simulink library "csc_snp_sensor_prep_lib"  (R2015b)
settings: Solver=ode45  SolverMode=SingleTasking  StartTime=0.0  StopTime=10.0  RelTol=1e-3
values from neighbouring files (symbols this model uses):
  snp_dtheta_filter_coeffs = fir1(snp_dtheta_filter_order,snp_dtheta_filter_freq)    [csc_snp_sensor_prep_init.m]
  snp_dtheta_filter_order = 1    [csc_snp_sensor_prep_init.m]
  snp_meas_noise_alt = [0.2 1000 1000]    [csc_snp_sensor_prep_init.m]
  snp_meas_noise_angle = 90.0    (= 90)    [csc_snp_sensor_prep_init.m]
  snp_meas_noise_angle_exp = 10    [csc_snp_sensor_prep_init.m]
  snp_meas_noise_angle_gain = 0.0    (= 0)    [csc_snp_sensor_prep_init.m]
  snp_meas_noise_dtheta = 4.0    (= 4)    [csc_snp_sensor_prep_init.m]
  snp_meas_noise_dtheta_exp = 11    [csc_snp_sensor_prep_init.m]
  snp_meas_noise_dtheta_gain = 0.0    (= 0)    [csc_snp_sensor_prep_init.m]
  snp_meas_noise_indep = [ 9e-4 9e-4 9e-4]    [csc_snp_sensor_prep_init.m]
  snp_R_lower_limit_alt = [0.001 10 10 ]    [csc_snp_sensor_prep_init.m]
  snp_R_lower_limit_angle = 0.0001    [csc_snp_sensor_prep_init.m]
  snp_R_lower_limit_dtheta = 0.0001    [csc_snp_sensor_prep_init.m]
  snp_zero_index = zeros(1,kfl_n_meas)    [csc_snp_sensor_prep_init.m]
  snp_zero_meas = zeros(kfl_n_meas,1)    [csc_snp_sensor_prep_init.m]
undefined symbols (not defined in the file or in its folder): kfl_topo_z_to_alt
libraries: simulink x4, util_info_lib x3, csc_hmg_homoraphy_meas_lib x3, csc_imu_sensor_prep_lib x3, csc_rsp_radar_sensor_prep_lib x3, csc_stg_tracker_sensor_prep_lib x3, csu_egm_estimated_gravity_model_lib x3
settings Model: ExtModeAutoUpdateStatusClock=off  Creator=Administrator  LastModifiedBy=Mark Agbayani
settings DataIOCC: SaveFormat=Array  SignalLoggingSaveFormat=ModelDataLogs
settings OptimizationCC: BlockReduction=off  BooleanDataType=off  ExpressionDepthLimit=2147483647
settings DebuggingCC: SaveWithParameterizedLinksMsg=none  UnderspecifiedInitializationDetection=Classic  MergeDetectMultiDrivingBlocksExec=none  SignalResolutionControl=TryResolveAllWithWarning  FcnCallInpInsideContextMsg=EnableAllAsWarning  StateNameClashWarn=warning  StrictBusMsg=Warning
settings HardwareCC: ProdBitPerPointer=32  ProdLargestAtomicFloat=None  ProdIntDivRoundTo=Undefined  ProdEndianess=Unspecified  ProdWordSize=32  ProdHWDeviceType=32-bit Generic  TargetUnknown=on
settings GRTTargetCC: GeneratePreprocessorConditionals=Disable all  CombineOutputUpdateFcns=off  GRTInterface=on
settings ConfigComp: CovModelRefEnable=Off  CovSFcnEnable=off

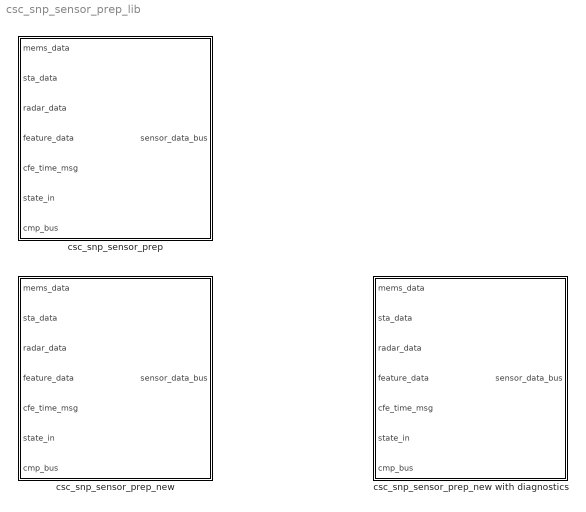
== system csc_snp_sensor_prep_lib ==
  csc_snp_sensor_prep : Subsystem
  csc_snp_sensor_prep_new : Subsystem
  csc_snp_sensor_prep_new with diagnostics : Subsystem  AncestorBlock=csc_snp_sensor_prep_lib/csc_snp_sensor_prep_new

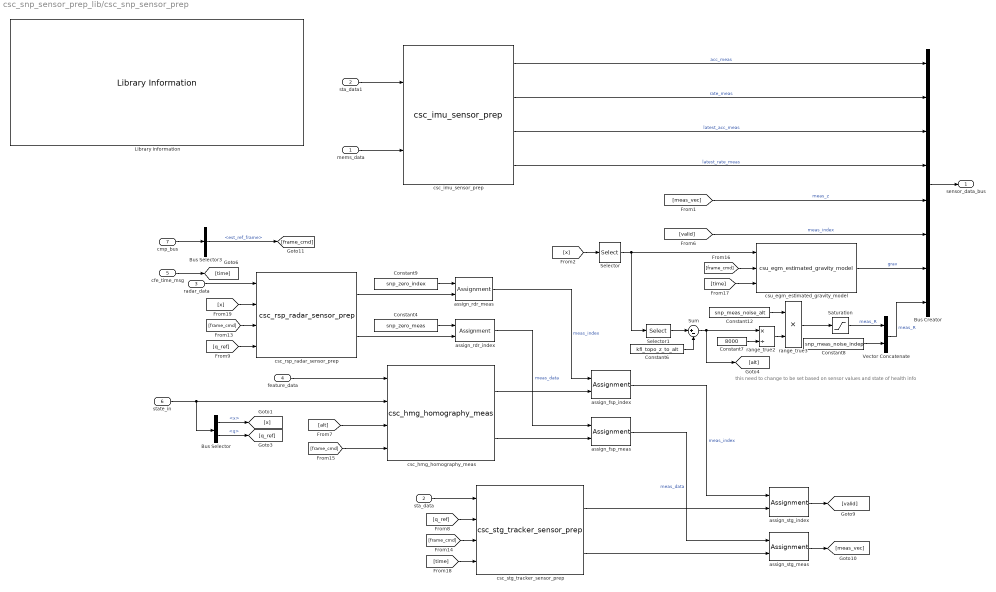
== system csc_snp_sensor_prep_lib/csc_snp_sensor_prep ==
  note: this need to change to be set based on sensor values and state of health info
  mems_data : Inport
  sta_data : Inport  Port=2
  radar_data : Inport  Port=3
  feature_data : Inport  Port=4
  cfe_time_msg : Inport  Port=5
  state_in : Inport  Port=6
  cmp_bus : Inport  Port=7
  Bus Creator : BusCreator  Inputs=8
  Bus Selector : BusSelector  OutputSignals=x,q
  Bus Selector3 : BusSelector  OutputSignals=est_ref_frame
  Constant12 : Constant  Value=snp_meas_noise_alt
  Constant4 : Constant  Value=snp_zero_meas
  Constant6 : Constant  Value=kfl_topo_z_to_alt
  Constant7 : Constant  Value=8000
  Constant8 : Constant  Value=snp_meas_noise_indep
  Constant9 : Constant  Value=snp_zero_index
  Library Information : util_info_lib/Library Information  owner='NONE'
  Saturation : Saturate  UpperLimit=1e20*[1 1 1]  LowerLimit=snp_R_lower_limit_alt
  Selector : Selector  InputPortWidth=kfl_n_state  IndexOptions=Index vector (dialog)  Indices=kfl_pos_index  OutputSizes=1
  Selector1 : Selector  InputPortWidth=3  IndexOptions=Index vector (dialog)  Indices=[3]  OutputSizes=1
  Sum : Sum  Inputs=|+-
  Vector Concatenate : Concatenate
  assign_fsp_index : Assignment  IndexOptions=Index vector (dialog)  Indices=snp_fsp_index  OutputSizes=1
  assign_fsp_meas : Assignment  IndexOptions=Index vector (dialog)  Indices=snp_fsp_index  OutputSizes=1
  assign_rdr_index : Assignment  IndexOptions=Index vector (dialog)  Indices=snp_rdr_index  OutputSizes=1
  assign_rdr_meas : Assignment  IndexOptions=Index vector (dialog)  Indices=snp_rdr_index  OutputSizes=1
  assign_stg_index : Assignment  IndexOptions=Index vector (dialog)  Indices=snp_stg_index  OutputSizes=1
  assign_stg_meas : Assignment  IndexOptions=Index vector (dialog)  Indices=snp_stg_index  OutputSizes=1
  csc_hmg_homography_meas : csc_hmg_homoraphy_meas_lib/csc_hmg_homography_meas
  csc_imu_sensor_prep : csc_imu_sensor_prep_lib/csc_imu_sensor_prep
  csc_rsp_radar_sensor_prep : csc_rsp_radar_sensor_prep_lib/csc_rsp_radar_sensor_prep
  csc_stg_tracker_sensor_prep : csc_stg_tracker_sensor_prep_lib/csc_stg_tracker_sensor_prep
  csu_egm_estimated_gravity_model : csu_egm_estimated_gravity_model_lib/csu_egm_estimated_gravity_model
  range_true2 : Product  Inputs=*/  RndMeth=Zero
  range_true3 : Product  RndMeth=Zero
  sta_data1 : InportShadow  Port=2
  sensor_data_bus : Outport
  wires:
  mems_data/1 -> csc_imu_sensor_prep/2
  sta_data1/1 -> csc_imu_sensor_prep/1
  csc_imu_sensor_prep/4 -> Bus Creator/4  "latest_rate_meas"
  csc_imu_sensor_prep/3 -> Bus Creator/3  "latest_acc_meas"
  csc_imu_sensor_prep/2 -> Bus Creator/2  "rate_meas"
  csc_imu_sensor_prep/1 -> Bus Creator/1  "acc_meas"
  csc_hmg_homography_meas/1 -> assign_fsp_index/2
  [q_ref] -> csc_rsp_radar_sensor_prep/4
  [alt] -> csc_hmg_homography_meas/3
  Constant9/1 -> assign_rdr_meas/1
  Constant4/1 -> assign_rdr_index/1
  csc_rsp_radar_sensor_prep/2 -> assign_rdr_index/2
  feature_data/1 -> csc_hmg_homography_meas/1
  [valid] -> Bus Creator/6  "meas_index"
  assign_rdr_meas/1 -> assign_fsp_index/1  "meas_index"
  assign_rdr_index/1 -> assign_fsp_meas/1  "meas_data"
  csc_hmg_homography_meas/2 -> assign_fsp_meas/2
  Bus Selector/1 -> [x]  "<x>"
  [x] -> Selector/1
  state_in/1 -> csc_hmg_homography_meas/2, Bus Selector/1
  csu_egm_estimated_gravity_model/1 -> Bus Creator/7  "grav"
  [meas_vec] -> Bus Creator/5  "meas_z"
  radar_data/1 -> csc_rsp_radar_sensor_prep/1
  csc_rsp_radar_sensor_prep/1 -> assign_rdr_meas/2
  Bus Creator/1 -> sensor_data_bus/1
  Selector/1 -> Selector1/1, csu_egm_estimated_gravity_model/1
  Constant6/1 -> Sum/2
  Selector1/1 -> Sum/1
  range_true2/1 -> range_true3/2
  Constant12/1 -> range_true3/1
  range_true3/1 -> Saturation/1
  cfe_time_msg/1 -> [time]
  Sum/1 -> range_true2/1, [alt]
  Constant7/1 -> range_true2/2
  sta_data/1 -> csc_stg_tracker_sensor_prep/1
  Bus Selector/2 -> [q_ref]  "<q>"
  [q_ref] -> csc_stg_tracker_sensor_prep/2
  [x] -> csc_rsp_radar_sensor_prep/2
  assign_fsp_index/1 -> assign_stg_index/1  "meas_index"
  assign_stg_index/1 -> [valid]
  assign_stg_meas/1 -> [meas_vec]
  assign_fsp_meas/1 -> assign_stg_meas/1  "meas_data"
  csc_stg_tracker_sensor_prep/2 -> assign_stg_meas/2
  csc_stg_tracker_sensor_prep/1 -> assign_stg_index/2
  cmp_bus/1 -> Bus Selector3/1
  [frame_cmd] -> csc_rsp_radar_sensor_prep/3
  [frame_cmd] -> csc_stg_tracker_sensor_prep/3
  [frame_cmd] -> csc_hmg_homography_meas/4
  [frame_cmd] -> csu_egm_estimated_gravity_model/2
  [time] -> csu_egm_estimated_gravity_model/3
  Bus Selector3/1 -> [frame_cmd]  "<est_ref_frame>"
  Saturation/1 -> Vector Concatenate/1  "meas_R"
  Vector Concatenate/1 -> Bus Creator/8  "meas_R"
  Constant8/1 -> Vector Concatenate/2
  [time] -> csc_stg_tracker_sensor_prep/4

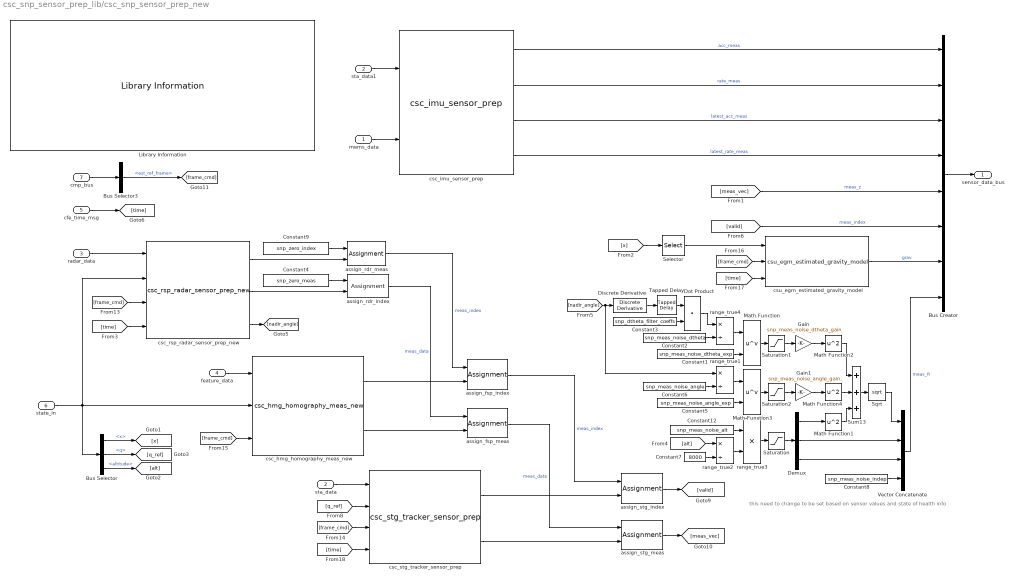
== system csc_snp_sensor_prep_lib/csc_snp_sensor_prep_new ==
  note: this need to change to be set based on sensor values and state of health info
  mems_data : Inport
  sta_data : Inport  Port=2
  radar_data : Inport  Port=3
  feature_data : Inport  Port=4
  cfe_time_msg : Inport  Port=5
  state_in : Inport  Port=6
  cmp_bus : Inport  Port=7
  Bus Creator : BusCreator  Inputs=8
  Bus Selector : BusSelector  OutputSignals=x,q,altitude
  Bus Selector3 : BusSelector  OutputSignals=est_ref_frame
  Constant1 : Constant  Value=snp_meas_noise_dtheta_exp
  Constant12 : Constant  Value=snp_meas_noise_alt
  Constant2 : Constant  Value=snp_meas_noise_dtheta
  Constant3 : Constant  Value=snp_dtheta_filter_coeffs
  Constant4 : Constant  Value=snp_zero_meas
  Constant5 : Constant  Value=snp_meas_noise_angle_exp
  Constant6 : Constant  Value=snp_meas_noise_angle
  Constant7 : Constant  Value=8000
  Constant8 : Constant  Value=snp_meas_noise_indep
  Constant9 : Constant  Value=snp_zero_index
  Demux : Demux  Outputs=3
  Discrete Derivative : simulink/Discrete/Discrete Derivative  gainval=1.0  ICPrevScaledInput=0.0  InputProcessing=Inherited  OutMin=[]  OutMax=[]  OutDataType=fixdt(1, 16)  OutScaling=2^-10  DoSatur=off
  Dot Product : DotProduct  InputSameDT=on  OutDataTypeStr=Inherit: Inherit via internal rule
  Gain : Gain  Gain=snp_meas_noise_dtheta_gain
  Gain1 : Gain  Gain=snp_meas_noise_angle_gain
  Library Information : util_info_lib/Library Information  owner='NONE'
  Math Function : Math  Operator=pow  SaturateOnIntegerOverflow=on
  Math Function1 : Math  Operator=square  SaturateOnIntegerOverflow=on
  Math Function2 : Math  Operator=square  SaturateOnIntegerOverflow=on
  Math Function3 : Math  Operator=pow  SaturateOnIntegerOverflow=on
  Math Function4 : Math  Operator=square  SaturateOnIntegerOverflow=on
  Saturation : Saturate  UpperLimit=1e20*[1 1 1]  LowerLimit=snp_R_lower_limit_alt
  Saturation1 : Saturate  UpperLimit=1e20  LowerLimit=snp_R_lower_limit_dtheta
  Saturation2 : Saturate  UpperLimit=1e20  LowerLimit=snp_R_lower_limit_angle
  Selector : Selector  InputPortWidth=kfl_n_state  IndexOptions=Index vector (dialog)  Indices=kfl_pos_index  OutputSizes=1
  Sqrt : Sqrt  SaturateOnIntegerOverflow=on
  Sum13 : Sum  Inputs=+++
  Tapped Delay : simulink/Discrete/Tapped Delay  vinit=0.0  samptime=-1  NumDelays=snp_dtheta_filter_order  DelayOrder=Oldest  includeCurrent=on
  Vector Concatenate : Concatenate  NumInputs=4
  assign_fsp_index : Assignment  IndexOptions=Index vector (dialog)  Indices=snp_fsp_index  OutputSizes=1
  assign_fsp_meas : Assignment  IndexOptions=Index vector (dialog)  Indices=snp_fsp_index  OutputSizes=1
  assign_rdr_index : Assignment  IndexOptions=Index vector (dialog)  Indices=snp_rdr_index  OutputSizes=1
  assign_rdr_meas : Assignment  IndexOptions=Index vector (dialog)  Indices=snp_rdr_index  OutputSizes=1
  assign_stg_index : Assignment  IndexOptions=Index vector (dialog)  Indices=snp_stg_index  OutputSizes=1
  assign_stg_meas : Assignment  IndexOptions=Index vector (dialog)  Indices=snp_stg_index  OutputSizes=1
  csc_hmg_homography_meas_new : csc_hmg_homoraphy_meas_lib/csc_hmg_homography_meas_new
  csc_imu_sensor_prep : csc_imu_sensor_prep_lib/csc_imu_sensor_prep
  csc_rsp_radar_sensor_prep_new : csc_rsp_radar_sensor_prep_lib/csc_rsp_radar_sensor_prep_new
  csc_stg_tracker_sensor_prep : csc_stg_tracker_sensor_prep_lib/csc_stg_tracker_sensor_prep
  csu_egm_estimated_gravity_model : csu_egm_estimated_gravity_model_lib/csu_egm_estimated_gravity_model
  range_true1 : Product  Inputs=*/  RndMeth=Zero
  range_true2 : Product  Inputs=*/  RndMeth=Zero
  range_true3 : Product  RndMeth=Zero
  range_true4 : Product  Inputs=*/  RndMeth=Zero
  sta_data1 : InportShadow  Port=2
  sensor_data_bus : Outport
  wires:
  Constant5/1 -> Math Function3/2
  Gain1/1 -> Math Function4/1
  Gain/1 -> Math Function2/1
  Math Function4/1 -> Sum13/2
  [nadir_angle] -> Discrete Derivative/1, range_true1/1
  Constant6/1 -> range_true1/2
  Constant1/1 -> Math Function/2
  range_true1/1 -> Math Function3/1
  Math Function3/1 -> Saturation2/1
  Saturation2/1 -> Gain1/1
  Discrete Derivative/1 -> Tapped Delay/1
  Constant3/1 -> Dot Product/2
  Tapped Delay/1 -> Dot Product/1
  Math Function1/1 -> Sum13/3
  Math Function2/1 -> Sum13/1
  Sqrt/1 -> Vector Concatenate/1
  Sum13/1 -> Sqrt/1
  Dot Product/1 -> range_true4/1
  Constant2/1 -> range_true4/2
  csc_rsp_radar_sensor_prep_new/3 -> [nadir_angle]
  range_true4/1 -> Math Function/1
  Math Function/1 -> Saturation1/1
  Saturation1/1 -> Gain/1
  Demux/1 -> Math Function1/1
  Demux/2 -> Vector Concatenate/2
  Demux/3 -> Vector Concatenate/3
  Bus Selector/3 -> [alt]  "<altitude>"
  [time] -> csc_rsp_radar_sensor_prep_new/4
  mems_data/1 -> csc_imu_sensor_prep/2
  sta_data1/1 -> csc_imu_sensor_prep/1
  csc_imu_sensor_prep/4 -> Bus Creator/4  "latest_rate_meas"
  csc_imu_sensor_prep/3 -> Bus Creator/3  "latest_acc_meas"
  csc_imu_sensor_prep/2 -> Bus Creator/2  "rate_meas"
  csc_imu_sensor_prep/1 -> Bus Creator/1  "acc_meas"
  csc_hmg_homography_meas_new/1 -> assign_fsp_index/2
  Constant9/1 -> assign_rdr_meas/1
  Constant4/1 -> assign_rdr_index/1
  csc_rsp_radar_sensor_prep_new/2 -> assign_rdr_index/2
  feature_data/1 -> csc_hmg_homography_meas_new/1
  [valid] -> Bus Creator/6  "meas_index"
  assign_rdr_meas/1 -> assign_fsp_index/1  "meas_index"
  assign_rdr_index/1 -> assign_fsp_meas/1  "meas_data"
  csc_hmg_homography_meas_new/2 -> assign_fsp_meas/2
  Bus Selector/1 -> [x]  "<x>"
  [x] -> Selector/1
  state_in/1 -> csc_rsp_radar_sensor_prep_new/2, csc_hmg_homography_meas_new/2, Bus Selector/1
  csu_egm_estimated_gravity_model/1 -> Bus Creator/7  "grav"
  [meas_vec] -> Bus Creator/5  "meas_z"
  radar_data/1 -> csc_rsp_radar_sensor_prep_new/1
  csc_rsp_radar_sensor_prep_new/1 -> assign_rdr_meas/2
  Bus Creator/1 -> sensor_data_bus/1
  Selector/1 -> csu_egm_estimated_gravity_model/1
  range_true2/1 -> range_true3/2
  Constant12/1 -> range_true3/1
  range_true3/1 -> Saturation/1
  cfe_time_msg/1 -> [time]
  [alt] -> range_true2/1
  Constant7/1 -> range_true2/2
  sta_data/1 -> csc_stg_tracker_sensor_prep/1
  Bus Selector/2 -> [q_ref]  "<q>"
  [q_ref] -> csc_stg_tracker_sensor_prep/2
  assign_fsp_index/1 -> assign_stg_index/1  "meas_index"
  assign_stg_index/1 -> [valid]
  assign_stg_meas/1 -> [meas_vec]
  assign_fsp_meas/1 -> assign_stg_meas/1  "meas_data"
  csc_stg_tracker_sensor_prep/2 -> assign_stg_meas/2
  csc_stg_tracker_sensor_prep/1 -> assign_stg_index/2
  cmp_bus/1 -> Bus Selector3/1
  [frame_cmd] -> csc_rsp_radar_sensor_prep_new/3
  [frame_cmd] -> csc_stg_tracker_sensor_prep/3
  [frame_cmd] -> csc_hmg_homography_meas_new/3
  [frame_cmd] -> csu_egm_estimated_gravity_model/2
  [time] -> csu_egm_estimated_gravity_model/3
  Bus Selector3/1 -> [frame_cmd]  "<est_ref_frame>"
  Saturation/1 -> Demux/1
  Vector Concatenate/1 -> Bus Creator/8  "meas_R"
  Constant8/1 -> Vector Concatenate/4
  [time] -> csc_stg_tracker_sensor_prep/4

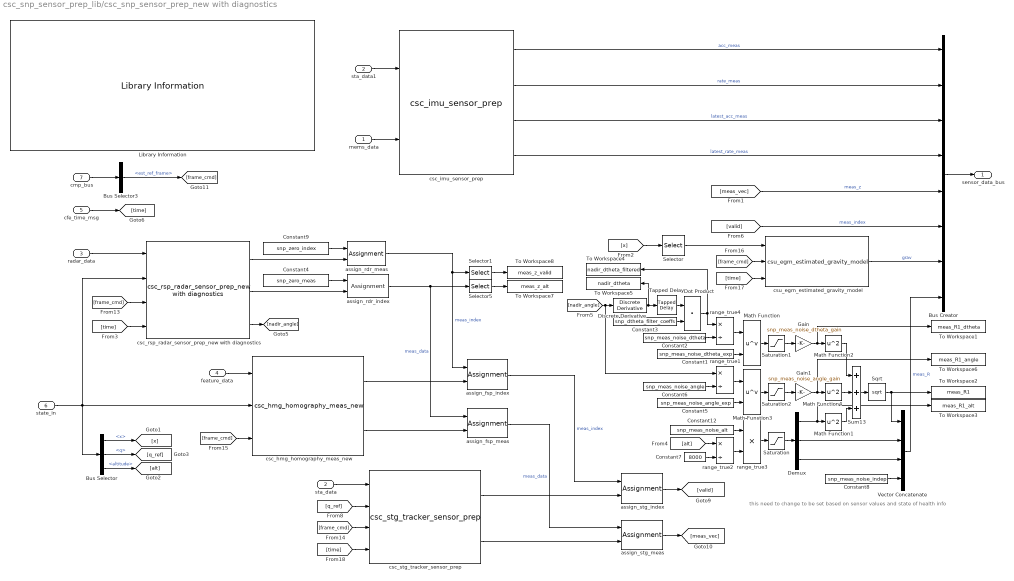
== system csc_snp_sensor_prep_lib/csc_snp_sensor_prep_new with diagnostics ==
  note: this need to change to be set based on sensor values and state of health info
  mems_data : Inport
  sta_data : Inport  Port=2
  radar_data : Inport  Port=3
  feature_data : Inport  Port=4
  cfe_time_msg : Inport  Port=5
  state_in : Inport  Port=6
  cmp_bus : Inport  Port=7
  Bus Creator : BusCreator  Inputs=8
  Bus Selector : BusSelector  OutputSignals=x,q,altitude
  Bus Selector3 : BusSelector  OutputSignals=est_ref_frame
  Constant1 : Constant  Value=snp_meas_noise_dtheta_exp
  Constant12 : Constant  Value=snp_meas_noise_alt
  Constant2 : Constant  Value=snp_meas_noise_dtheta
  Constant3 : Constant  Value=snp_dtheta_filter_coeffs
  Constant4 : Constant  Value=snp_zero_meas
  Constant5 : Constant  Value=snp_meas_noise_angle_exp
  Constant6 : Constant  Value=snp_meas_noise_angle
  Constant7 : Constant  Value=8000
  Constant8 : Constant  Value=snp_meas_noise_indep
  Constant9 : Constant  Value=snp_zero_index
  Demux : Demux  Outputs=3
  Discrete Derivative : simulink/Discrete/Discrete Derivative  gainval=1.0  ICPrevScaledInput=0.0  InputProcessing=Inherited  OutMin=[]  OutMax=[]  OutDataType=fixdt(1, 16)  OutScaling=2^-10  DoSatur=off
  Dot Product : DotProduct  InputSameDT=on  OutDataTypeStr=Inherit: Inherit via internal rule
  Gain : Gain  Gain=snp_meas_noise_dtheta_gain
  Gain1 : Gain  Gain=snp_meas_noise_angle_gain
  Library Information : util_info_lib/Library Information  owner='NONE'
  Math Function : Math  Operator=pow  SaturateOnIntegerOverflow=on
  Math Function1 : Math  Operator=square  SaturateOnIntegerOverflow=on
  Math Function2 : Math  Operator=square  SaturateOnIntegerOverflow=on
  Math Function3 : Math  Operator=pow  SaturateOnIntegerOverflow=on
  Math Function4 : Math  Operator=square  SaturateOnIntegerOverflow=on
  Saturation : Saturate  UpperLimit=1e20*[1 1 1]  LowerLimit=snp_R_lower_limit_alt
  Saturation1 : Saturate  UpperLimit=1e20  LowerLimit=snp_R_lower_limit_dtheta
  Saturation2 : Saturate  UpperLimit=1e20  LowerLimit=snp_R_lower_limit_angle
  Selector : Selector  InputPortWidth=kfl_n_state  IndexOptions=Index vector (dialog)  Indices=kfl_pos_index  OutputSizes=1
  Selector1 : Selector  InputPortWidth=kfl_n_meas  IndexOptions=Index vector (dialog)  Indices=snp_rdr_index  OutputSizes=1
  Selector5 : Selector  InputPortWidth=kfl_n_meas  IndexOptions=Index vector (dialog)  Indices=snp_rdr_index  OutputSizes=1
  Sqrt : Sqrt  SaturateOnIntegerOverflow=on
  Sum13 : Sum  Inputs=+++
  Tapped Delay : simulink/Discrete/Tapped Delay  vinit=0.0  samptime=-1  NumDelays=snp_dtheta_filter_order  DelayOrder=Oldest  includeCurrent=on
  To Workspace1 : ToWorkspace  VariableName=meas_R1_dtheta  SaveFormat=Structure With Time  SampleTime=-1
  To Workspace2 : ToWorkspace  VariableName=meas_R1  SaveFormat=Structure With Time  SampleTime=-1
  To Workspace3 : ToWorkspace  VariableName=meas_R1_alt  SaveFormat=Structure With Time  SampleTime=-1
  To Workspace4 : ToWorkspace  VariableName=nadir_dtheta_filtered  SaveFormat=Structure With Time  SampleTime=-1
  To Workspace5 : ToWorkspace  VariableName=nadir_dtheta  SaveFormat=Structure With Time  SampleTime=-1
  To Workspace6 : ToWorkspace  VariableName=meas_R1_angle  SaveFormat=Structure With Time  SampleTime=-1
  To Workspace7 : ToWorkspace  VariableName=meas_z_alt  SaveFormat=Structure With Time  SampleTime=-1
  To Workspace8 : ToWorkspace  VariableName=meas_z_valid  SaveFormat=Structure With Time  SampleTime=-1
  Vector Concatenate : Concatenate  NumInputs=4
  assign_fsp_index : Assignment  IndexOptions=Index vector (dialog)  Indices=snp_fsp_index  OutputSizes=1
  assign_fsp_meas : Assignment  IndexOptions=Index vector (dialog)  Indices=snp_fsp_index  OutputSizes=1
  assign_rdr_index : Assignment  IndexOptions=Index vector (dialog)  Indices=snp_rdr_index  OutputSizes=1
  assign_rdr_meas : Assignment  IndexOptions=Index vector (dialog)  Indices=snp_rdr_index  OutputSizes=1
  assign_stg_index : Assignment  IndexOptions=Index vector (dialog)  Indices=snp_stg_index  OutputSizes=1
  assign_stg_meas : Assignment  IndexOptions=Index vector (dialog)  Indices=snp_stg_index  OutputSizes=1
  csc_hmg_homography_meas_new : csc_hmg_homoraphy_meas_lib/csc_hmg_homography_meas_new
  csc_imu_sensor_prep : csc_imu_sensor_prep_lib/csc_imu_sensor_prep
  csc_rsp_radar_sensor_prep_new with diagnostics : csc_rsp_radar_sensor_prep_lib/csc_rsp_radar_sensor_prep_new with diagnostics
  csc_stg_tracker_sensor_prep : csc_stg_tracker_sensor_prep_lib/csc_stg_tracker_sensor_prep
  csu_egm_estimated_gravity_model : csu_egm_estimated_gravity_model_lib/csu_egm_estimated_gravity_model
  range_true1 : Product  Inputs=*/  RndMeth=Zero
  range_true2 : Product  Inputs=*/  RndMeth=Zero
  range_true3 : Product  RndMeth=Zero
  range_true4 : Product  Inputs=*/  RndMeth=Zero
  sta_data1 : InportShadow  Port=2
  sensor_data_bus : Outport
  wires:
  [time] -> csc_stg_tracker_sensor_prep/4
  Constant8/1 -> Vector Concatenate/4
  Vector Concatenate/1 -> Bus Creator/8  "meas_R"
  Saturation/1 -> Demux/1
  Bus Selector3/1 -> [frame_cmd]  "<est_ref_frame>"
  [time] -> csu_egm_estimated_gravity_model/3
  [frame_cmd] -> csu_egm_estimated_gravity_model/2
  [frame_cmd] -> csc_hmg_homography_meas_new/3
  [frame_cmd] -> csc_stg_tracker_sensor_prep/3
  [frame_cmd] -> csc_rsp_radar_sensor_prep_new with diagnostics/3
  cmp_bus/1 -> Bus Selector3/1
  csc_stg_tracker_sensor_prep/1 -> assign_stg_index/2
  csc_stg_tracker_sensor_prep/2 -> assign_stg_meas/2
  assign_fsp_meas/1 -> assign_stg_meas/1  "meas_data"
  assign_stg_meas/1 -> [meas_vec]
  assign_stg_index/1 -> [valid]
  assign_fsp_index/1 -> assign_stg_index/1  "meas_index"
  [q_ref] -> csc_stg_tracker_sensor_prep/2
  Bus Selector/2 -> [q_ref]  "<q>"
  sta_data/1 -> csc_stg_tracker_sensor_prep/1
  Constant7/1 -> range_true2/2
  [alt] -> range_true2/1
  cfe_time_msg/1 -> [time]
  range_true3/1 -> Saturation/1
  Constant12/1 -> range_true3/1
  range_true2/1 -> range_true3/2
  Selector/1 -> csu_egm_estimated_gravity_model/1
  Bus Creator/1 -> sensor_data_bus/1
  csc_rsp_radar_sensor_prep_new with diagnostics/1 -> assign_rdr_meas/2
  radar_data/1 -> csc_rsp_radar_sensor_prep_new with diagnostics/1
  [meas_vec] -> Bus Creator/5  "meas_z"
  csu_egm_estimated_gravity_model/1 -> Bus Creator/7  "grav"
  state_in/1 -> csc_rsp_radar_sensor_prep_new with diagnostics/2, csc_hmg_homography_meas_new/2, Bus Selector/1
  [x] -> Selector/1
  Bus Selector/1 -> [x]  "<x>"
  csc_hmg_homography_meas_new/2 -> assign_fsp_meas/2
  assign_rdr_index/1 -> Selector5/1, assign_fsp_meas/1  "meas_data"
  assign_rdr_meas/1 -> Selector1/1, assign_fsp_index/1  "meas_index"
  [valid] -> Bus Creator/6  "meas_index"
  feature_data/1 -> csc_hmg_homography_meas_new/1
  csc_rsp_radar_sensor_prep_new with diagnostics/2 -> assign_rdr_index/2
  Constant4/1 -> assign_rdr_index/1
  Constant9/1 -> assign_rdr_meas/1
  csc_hmg_homography_meas_new/1 -> assign_fsp_index/2
  csc_imu_sensor_prep/1 -> Bus Creator/1  "acc_meas"
  csc_imu_sensor_prep/2 -> Bus Creator/2  "rate_meas"
  csc_imu_sensor_prep/3 -> Bus Creator/3  "latest_acc_meas"
  csc_imu_sensor_prep/4 -> Bus Creator/4  "latest_rate_meas"
  sta_data1/1 -> csc_imu_sensor_prep/1
  mems_data/1 -> csc_imu_sensor_prep/2
  [time] -> csc_rsp_radar_sensor_prep_new with diagnostics/4
  Bus Selector/3 -> [alt]  "<altitude>"
  Demux/3 -> Vector Concatenate/3
  Demux/2 -> Vector Concatenate/2
  Saturation1/1 -> Gain/1
  Math Function/1 -> Saturation1/1
  range_true4/1 -> Math Function/1
  csc_rsp_radar_sensor_prep_new with diagnostics/3 -> [nadir_angle]
  Constant2/1 -> range_true4/2
  Sum13/1 -> Sqrt/1
  Math Function2/1 -> Sum13/1
  Math Function1/1 -> Sum13/3
  Tapped Delay/1 -> Dot Product/1
  Constant3/1 -> Dot Product/2
  Saturation2/1 -> Gain1/1
  Math Function3/1 -> Saturation2/1
  range_true1/1 -> Math Function3/1
  Constant1/1 -> Math Function/2
  Constant6/1 -> range_true1/2
  [nadir_angle] -> range_true1/1, Discrete Derivative/1
  Math Function4/1 -> Sum13/2
  Constant5/1 -> Math Function3/2
  Selector1/1 -> To Workspace8/1
  Selector5/1 -> To Workspace7/1
  Gain1/1 -> To Workspace6/1, Math Function4/1
  Gain/1 -> To Workspace1/1, Math Function2/1
  Discrete Derivative/1 -> To Workspace5/1, Tapped Delay/1
  Sqrt/1 -> To Workspace2/1, Vector Concatenate/1
  Dot Product/1 -> To Workspace4/1, range_true4/1
  Demux/1 -> To Workspace3/1, Math Function1/1
